simulink model "WInd_Power_Simulation"  (R2024b)
settings: Solver=VariableStepAuto  StartTime=0.0  StopTime=10.0  RelTol=1e-3
settings Model: Creator=jayesh sunil gurav  LastModifiedBy=amolg
settings OptimizationCC: ReuseModelBlockBuffer=off
settings DebuggingCC: UnconnectedInputMsg=warning  UnconnectedOutputMsg=warning  UnconnectedLineMsg=warning
settings ModelReferenceCC: EnableRefExpFcnMdlSchedulingChecks=on
settings RTWCC: GPUComputeCapability=3.5  DLArmComputeVersion=19.05

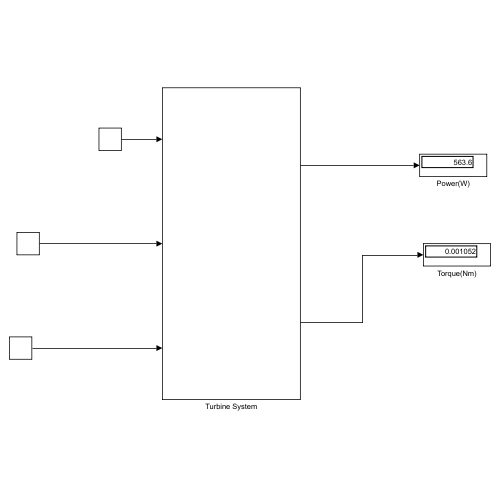
[thumbnail: Simulink's stored preview of the top-level diagram]
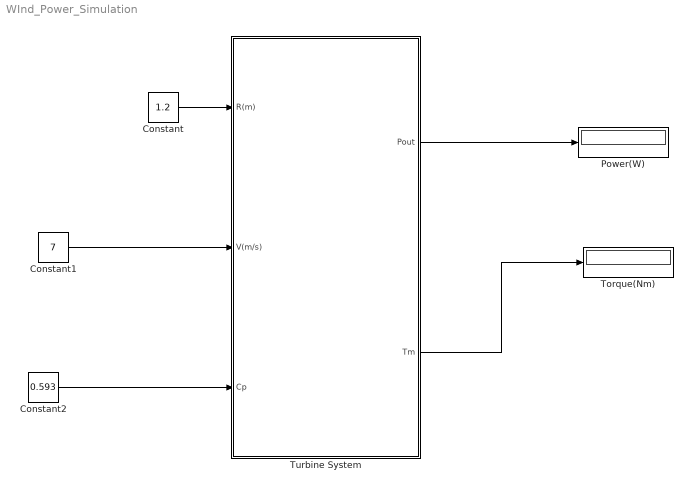
== system WInd_Power_Simulation ==
  Constant : Constant  Value=1.2
  Constant1 : Constant  Value=7
  Constant2 : Constant  Value=0.593
  Power(W) : Display
  Torque(Nm) : Display
  Turbine System : Subsystem
  wires:
  Constant/1 -> Turbine System/1(R(m))
  Constant1/1 -> Turbine System/2(V(m/s))
  Constant2/1 -> Turbine System/3(Cp)
  Turbine System/1(Pout) -> Power(W)/1
  Turbine System/2(Tm) -> Torque(Nm)/1

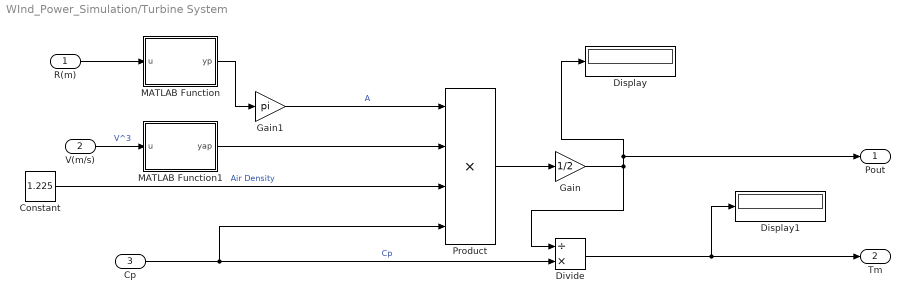
== system WInd_Power_Simulation/Turbine System ==
  R(m) : Inport
  V(m/s) : Inport  Port=2
  Cp : Inport  Port=3
  Constant : Constant  Value=1.225
  Display : Display
  Display1 : Display
  Divide : Product  Inputs=/*
  Gain : Gain  Gain=1/2
  Gain1 : Gain  Gain=pi
  MATLAB Function : MATLAB Function  TreatAsAtomicUnit=on
  MATLAB Function1 : MATLAB Function  TreatAsAtomicUnit=on
  Product : Product  Inputs=4
  Pout : Outport
  Tm : Outport  Port=2
  wires:
  Product/1 -> Gain/1
  Gain1/1 -> Product/1  "A"
  V(m/s)/1 -> MATLAB Function1/1(u)  "V^3"
  Constant/1 -> Product/3  "Air Density"
  Cp/1 -> Product/4, Divide/2  "Cp"
  R(m)/1 -> MATLAB Function/1(u)
  Gain/1 -> Divide/1, Display/1, Pout/1
  Divide/1 -> Tm/1, Display1/1
  MATLAB Function/1(yp) -> Gain1/1
  MATLAB Function1/1(yap) -> Product/2

== matlab function WInd_Power_Simulation/Turbine System/MATLAB Function ==
  data: u input; yp output
function yp = fcn(u)

yp = u^2;
end

== matlab function WInd_Power_Simulation/Turbine System/MATLAB Function1 ==
  data: u input; yap output
function yap = fcn(u)

yap = u^3;
end
